simulink library "c166drivers"  (Simulink 6.0)
settings: Solver=ode45  SolverMode=SingleTasking  StartTime=0.0  StopTime=10.0  RelTol=1e-3
PreLoadFcn:
  | RTWConfigurationCB('preloadfcn', bdroot);
libraries: c166drivers x12, canblocks x8, exprofilelib x6, config_library x4, driver_interface_library x4, canblocks_extras x4, vector_candrivers x2, simulink x1
settings Model: Creator=The MathWorks Inc.  LastModifiedBy=batserve  ExtModeAutoUpdateStatusClock=off  ProdHWDeviceType=Specified
settings DataIOCC: SignalLoggingName=logsOut
settings OptimizationCC: BooleanDataType=off
settings DebuggingCC: CheckExecutionContextPreStartOutputMsg=on  CheckExecutionContextRuntimeOutputMsg=on  SolverPrmCheckMsg=none
settings HardwareCC: ProdHWDeviceType=Specified  TargetUnknown=on

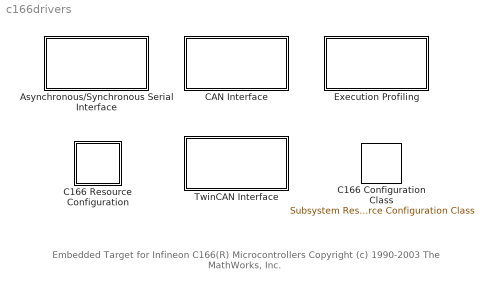
== system c166drivers ==
  note: Embedded Target for Infineon C166(R) Microcontrollers
      | Copyright (c) 1990-2003 The MathWorks, Inc.
  Asynchronous/Synchronous Serial Interface : Subsystem  PropExecContextAcrossSSBoundary=on
      mask Display: disp('Serial')
  C166 Configuration Class : config_library/Subsystem Resource Configuration Class  Tag=CONFIGURATION DATA CLASS  dClassName=c166Config.C166System  rClassName=c166Config.C166SystemResources
  C166 Resource Configuration : Subsystem  Tag=RTW CONFIGURATION BLOCK  AncestorBlock=|  PropExecContextAcrossSSBoundary=on  mask(Subsystem Resource Configuration){oldParentName=untitled2, oldBlockName=|, defaultConfigLibrary=}
      | config_library/Subsystem
      | Resource
      | Configuration
      mask oldBlockName=|
      | untitled2/C166
      | Resource
      | Configuration
      mask prompts: oldParentName "Old Parent Name"; oldBlockName "Old Block Name"; defaultConfigLibrary "Default Configuration Library"
      settings: CopyFcn=RTWConfigurationCB('copyfcn',gcb);  DeleteFcn=RTWConfigurationCB('deletefcn',gcb);  UndoDeleteFcn=RTWConfigurationCB('NameChangeFcn',gcb);  PreSaveFcn=RTWConfigurationCB('presavefcn',gcb);  NameChangeFcn=RTWConfigurationCB('NameChangeFcn',gcb);  OpenFcn=RTWConfigurationCB('openfcn',gcb);
      mask Display: image(imread('target_icon.jpg'))
  CAN Interface : Subsystem  PropExecContextAcrossSSBoundary=on
      mask Display: disp('CAN')
  Execution Profiling : Subsystem  PropExecContextAcrossSSBoundary=on
      mask Display: disp('Execution\nProfiling')
  TwinCAN Interface : Subsystem  PropExecContextAcrossSSBoundary=on
      mask Display: disp('TwinCAN')

== system c166drivers/Asynchronous/Synchronous Serial Interface ==
  ASC_Serial Configuration Class : config_library/Subsystem Resource Configuration Class  Tag=CONFIGURATION DATA CLASS  dClassName=c166Config.ASC_SERIAL  rClassName=""
  Serial Receive : S-Function  FunctionName=asc0_rx  Parameters=T,show_length,show_bytes_read, max_length  mask(C166 Serial Interface ASC0 Receive){show_length=on, show_bytes_read=on, max_length=1, T=1}
      mask prompts: show_length "Show input port for the requested number of bytes"; show_bytes_read "Show output port for the actual number of bytes read"; max_length "Maximum number of bytes:"; T "Sample time:"
      mask help: Receive bytes over the serial interface ASC0. Note that if the number of bytes available is smaller than the number of bytes requested then the actual number of bytes read is equal to the number of bytes available.
      mask init:
      | % Check for a C166 Resource Configuration block
      | target = RTWConfigurationCB('get_target', gcb);                            
      | target.checkName('C166');        
      | 
      | % Allocate the serial transmit interface
      | serial_interface = mask_resource_validator(gcb,@c166_serial_resource,'ASC0_RX');
      | if round(max_length)~=max_length | max_length<1
      | 	error('The maximum length of data parameter must be a positive integer')
      | end
      mask Help: helpview([docroot '/toolbox/c166/c166.map'], 'Serial_Receive');
      mask CallbackString:
      | s = get_param(gcb,'show_length');
      | if strcmp(s,'on')
      |    simUtil_maskParam('show',gcb,'max_length');
      | else
      |    simUtil_maskParam('hide',gcb,'max_length');
      | end
      | |||
      mask Display:
      | text(0.5, 0.5, 'ASC0\nReceive','horizontalAlignment','center')
      | port_label('output',1,'Data')
  Serial Transmit : S-Function  FunctionName=asc0_tx  Parameters=T,show_length,show_num_sent  mask(C166 Serial Interface ASC0 Transmit){show_length=on, show_num_sent=on, T=-1}
      mask prompts: show_length "Show input port for the number of bytes to transmit"; show_num_sent "Show output port for the actual number of bytes transmitted"; T "Sample time:"
      mask help: Transmit bytes over the serial interface ASC0. Note that if the number of available spaces in the buffer is smaller than the requested number of bytes to transmit then the actual number of bytes transmitted is equal to the number of spaces available.
      mask init:
      | % Check for a C166 Resource Configuration block
      | target = RTWConfigurationCB('get_target', gcb);                            
      | target.checkName('C166');        
      | 
      | % Allocate the serial transmit interface
      | serial_interface = mask_resource_validator(gcb,@c166_serial_resource,'ASC0_TX');
      mask Help: helpview([docroot '/toolbox/c166/c166.map'], 'Serial_Transmit');
      mask Display:
      | text(0.5, 0.5, 'ASC0\nTransmit','horizontalAlignment','center')
      | port_label('input',1,'Data')

== system c166drivers/C166 Resource Configuration ==
  config : S-Function  FunctionName=sfunRTWConfig

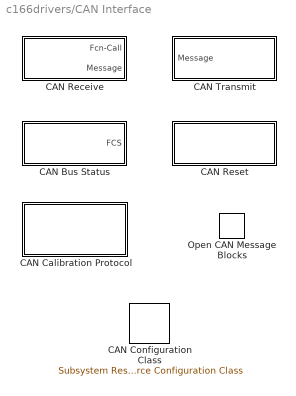
== system c166drivers/CAN Interface ==
  CAN Configuration Class : config_library/Subsystem Resource Configuration Class  Tag=CONFIGURATION DATA CLASS  dClassName=c166Config.CAN_C166  rClassName=c166Config.CAN_RESOURCES
  CAN Bus Status : Subsystem  PropExecContextAcrossSSBoundary=on  mask(C166 CAN Bus Status){module=A, status_type=Bus Off, t=1}
      mask prompts: status_type "Status type:"; t "Sample time:"
      mask help: Use this block to determine if the CAN controller is in either Bus Off state or Error Warning state.
      mask init:
      | dispstr = sprintf('CAN_%s\n%s Status', get_param(gcb,'module'),get_param(gcb,'status_type'));
      | 
      | % Check for a C166 Resource Configuration block
      | target = RTWConfigurationCB('get_target', gcb);                            
      | target.checkName('C166');        
      | 
      | if status_type == 1
      | 	status_str = 'Bus Off';
      | elseif status_type == 2
      | 	status_str = 'Error Warning';
      | end
      mask Help: helpview([docroot '/toolbox/c166/c166.map'], 'CAN_bus_status');
      mask StyleString: popup(A|B),popup(Bus Off|Error Warning),edit
      mask Display: disp(dispstr)
  CAN Calibration Protocol : Subsystem  TreatAsAtomicUnit=on  PropExecContextAcrossSSBoundary=on  mask(CAN Calibration Protocol (C166)){CCP_STATION_ID=hex2dec('1'), module=A, ccp_cro_id=hex2dec('6FA'), ccp_cro_message_type=Extended (29-bit identifier), ccp_return_id=hex2dec('6FB'), ccp_return_message_type=Extended (29-bit identifier), TOTAL_NUM_ODTS=8, cro_sample_time=0.01}
      mask prompts: CCP_STATION_ID "CCP station address (16-bit integer):"; module "CAN module:"; ccp_cro_id "CAN message identifier (CRO):"; ccp_cro_message_type "CAN message type (CRO):"; ccp_return_id "CAN message identifier (DTO/DAQ):"; ccp_return_message_type "CAN message type (DTO/DAQ):"; TOTAL_NUM_ODTS "Total Number of Object Descriptor Tables (ODTs):"; cro_sample_time "CRO sample time:"
      mask help:
      | Implements CAN Calibration Protocol (CCP v2.1) on the target processor.
      |
      | This block processes Command Receive Object (CRO) messages and outputs the resulting Data Transmission Object (DTO) and Data Acquisition (DAQ) messages.
      mask init:
      | % Propagate DTO message type to underlying blocks
      | set_param([gcb, '/DAQ Processing/Send DAQ Message/CAN Message Packing'], 'message_type', ccp_return_message_type);
      | set_param([gcb, '/DTO Processing/CCP (Termination)/CAN Transmit/DTO_Constructor'], 'message_type', ccp_return_message_type);
      | % Propagate CRO message type to underlying blocks
      | set_param([gcb, '/CAN Receive'], 'message_type', ccp_cro_message_type);
      | % Propagate CAN module to underlying blocks
      | set_param([gcb, '/DAQ Processing/Send DAQ Message/CAN Transmit'], 'module', module);
      | set_param([gcb, '/DTO Processing/CCP (Termination)/CAN Transmit/CAN Transmit'], 'module', module);
      | set_param([gcb, '/CAN Receive'], 'module', module);
      | 
      | % check for a Resource Config block, and make sure it is C166
      | target = RTWConfigurationCB('get_target', gcb);
      | target.checkName('C166');
      settings: CopyFcn=ccp_init_mask('copyfcn', gcb)
      mask Help: helpview([docroot '/toolbox/c166/c166.map'], 'target_CCP');
      mask StyleString: edit,popup(A|B),edit,popup(Standard (11-bit identifier)|Extended (29-bit identifier)),edit,popup(Standard (11-bit identifier)|Extended (29-bit identifier)),edit,edit
      mask Display: disp('CCP');
  CAN Receive : Subsystem  PropExecContextAcrossSSBoundary=on  mask(C166 CAN Receive){module=A, ids=hex2dec('0001'), buffer_select_mode=Automatic, bufferids=1, message_type=Standard (11-bit identifier), t=1}
      mask prompts: module "CAN module:"; ids "CAN message identifier:"; buffer_select_mode "Buffer selection:"; bufferids "Buffer number [1..15]:"; message_type "CAN message type:"; t "Sample time:"
      mask help: Receives CAN messages from the selected CAN module.
      mask init:
      | dispstr = sprintf('CAN_%s\nReceive',get_param(gcb,'module'));
      | 
      | % Check for a C166 Resource Configuration block
      | target = RTWConfigurationCB('get_target', gcb);                            
      | target.checkName('C166');        
      | 
      | if any(bufferids>15) | any(bufferids<1) | any( ~[bufferids==fix(bufferids)] )
      | 	error('Invalid CAN hardware buffer number specified. The buffer number number must be an integer in the range 1 to 15');
      | end
      | 
      | % Possibly auto-allocate the buffer
      | bufferids = mask_resource_validator(gcb,@c166_can_rx_validate, bufferids);
      | 
      | % check for valid CAN message identifier
      | can_msg_id_check(ids,message_type);
      | message_type=message_type-1;
      | 
      | % Check that module is enabled
      | c166_can_enabled_check(gcb,'CAN');
      mask Help: helpview([docroot '/toolbox/c166/c166.map'], 'CAN_RX');
      mask StyleString: popup(A|B),edit,popup(Automatic|Manual),edit,popup(Standard (11-bit identifier)|Extended (29-bit identifier)),edit
      mask CallbackString:
      | ||switch get_param(gcb,'buffer_select_mode');
      | 	case 'Automatic'
      | 		simUtil_maskParam('disable',gcb,'bufferids');
      | 	case 'Manual'
      |          simUtil_maskParam('enable',gcb,'bufferids');
      |  end
      |  |||
      mask Display:
      | disp(dispstr)
      | port_label('output',1,'f()');
      | port_label('output',2,'Msg');
  CAN Reset : Subsystem  PropExecContextAcrossSSBoundary=on  mask(C166 CAN Reset){module=A, t=-1}
      mask prompts: t "Sample time:"
      mask help: Place this block inside a triggered sub-system to reset the CAN module, for example, following entry to the Bus Off state.
      mask init:
      | dispstr = sprintf('CAN_%s\nReset', get_param(gcb,'module'));
      | 
      | % Check for a C166 Resource Configuration block
      | target = RTWConfigurationCB('get_target', gcb);                            
      | target.checkName('C166');
      mask Help: helpview([docroot '/toolbox/c166/c166.map'], 'CAN_reset');
      mask StyleString: popup(A|B),edit
      mask Display: disp(dispstr)
  CAN Transmit : Subsystem  PropExecContextAcrossSSBoundary=on  mask(C166 CAN Transmit){module=A, tx_mode=Queued transmission with shared buffer, fifo_queue_length=8, buffer_select_mode=Automatic, bufferids=1, t=-1, irq_level=0}
      mask prompts: tx_mode "Transmit mode:"; fifo_queue_length "Length (number of messages) of FIFO queue:"; buffer_select_mode "Buffer selection:"; bufferids "Buffer number [1..14]:"; t "Sample time:"; irq_level "Interrupt level (hidden)"
      mask help: Transmits a CAN message via the selected CAN module.
      mask init:
      | dispstr=sprintf('CAN_%s\nTransmit', get_param(gcb,'module'));
      | 
      | % Check for a C166 Resource Configuration block
      | target = RTWConfigurationCB('get_target', gcb);                            
      | target.checkName('C166');        
      | 
      | if bufferids==0 % special handling for un-initialized value
      | 	bufferids=1;
      | end
      | 
      | if any(bufferids>14) | any(bufferids<1) | any( ~[bufferids==fix(bufferids)] )
      | 	error('Invalid CAN hardware buffer number specified. The buffer number number must be an integer in the range 1 to 14 (it is not possible to use buffer 15 for transmit).');
      | end
      | 
      | 
      | % Check that module is enabled
      | c166_can_enabled_check(gcb,'CAN');
      | 
      | % Possibly auto-allocate the buffer
      | bufferids = mask_resource_validator(gcb,@c166_can_tx_validate,bufferids);
      | 
      | irq_level = 0;
      | 
      |   switch tx_mode
      |    case 1
      |     % no action
      |    case 2
      |     % no action
      |    case 3
      |     CAN = target.findConfigForClass('c166Config.CAN_C166');
      | 	if module == 1
      |         CAN.CAN_A.RequireIntDrivenFifoTx = 1;
      | 		irq_level = str2num(CAN.CAN_A.CAN_interrupt_level);
      | 	elseif module == 2
      |         CAN.CAN_B.RequireIntDrivenFifoTx = 1;
      | 		irq_level = str2num(CAN.CAN_B.CAN_Interrupt_Level);
      | 	end
      |    otherwise
      |     error('Invalid value for tx_mode')
      |   end
      mask Help: helpview([docroot '/toolbox/c166/c166.map'], 'CAN_TX');
      mask StyleString: popup(A|B),popup(Queued transmission with shared buffer|Direct transmission with dedicated buffer|FIFO queued transmission with dedicated buffer),edit,popup(Automatic|Manual),edit,edit,edit
      mask CallbackString:
      | |tempCanTxTxMode = get_param(gcb,'tx_mode');
      | switch tempCanTxTxMode
      | 	case {'Queued transmission with shared buffer'}
      | 		simUtil_maskParam('hide',gcb,'fifo_queue_length');
      | 		simUtil_maskParam('hide',gcb,'buffer_select_mode');
      | 		simUtil_maskParam('hide',gcb,'bufferids');
      | 	case {'Direct transmission with dedicated buffer'}
      | 		simUtil_maskParam('hide',gcb,'fifo_queue_length');
      | 		simUtil_maskParam('show',gcb,'buffer_select_mode');
      | 		simUtil_maskParam('show',gcb,'bufferids');
      |     case 'FIFO queued transmission with dedicated buffer'
      | 	    simUtil_maskParam('show',gcb,'fifo_queue_length');
      | 		simUtil_maskParam('show',gcb,'buffer_select_mode');
      | 		simUtil_maskParam('show',gcb,'bufferids');
      | 	otherwise
      | 		error(['Unrecognized value for tx_mode in ' gcb ]);
      | end
      | clear tempCanTxTxMode||switch get_param(gcb,'buffer_select_mode');
      | 	case 'Automatic'
      | 		simUtil_maskParam('disable',gcb,'bufferids');
      | 	case 'Manual'
      |          simUtil_maskParam('enable',gcb,'bufferids');
      |  end
      |  |
      |  ||
      mask Display:
      | disp(dispstr)
      | port_label('input',1,'Msg');
  Open CAN Message Blocks : vector_candrivers/Open CAN Message Blocks

== system c166drivers/Execution Profiling ==
  C166 Execution Profiling via ASC0 : Subsystem  TreatAsAtomicUnit=on  PropExecContextAcrossSSBoundary=on  mask(C166  Execution Profiling via Serial Port ASC0){t=1, execCopyFcn=on}
      mask prompts: t "Sample time:"; execCopyFcn "Execute CopyFcn"
      mask help:
      | Provides a serial interface to the execution profiling engine. On receipt of a start command to the serial port, logging of execution profile data begins. On completion of a logging run, the recorded data is automatically returned via serial.
      |
      | No other serial blocks may be used in the model if a C166 Execution Profiling via ASC0 block is present.
      |
      | See also the MATLAB command profile_c166.
      settings: CopyFcn=exprofile_copyfcn(gcb);
      mask Help: helpview([docroot '/toolbox/c166/c166.map'], 'Execution_Profiling_ASC0');
      mask Display: disp('Execution Profiling\nvia Serial')
  C166 Execution Profiling via CAN A : Subsystem  TreatAsAtomicUnit=on  PropExecContextAcrossSSBoundary=on  mask(C166 Execution Profiling via CAN Channel A){commandId=hex2dec('1FFFFF00'), dataId=hex2dec('1FFFFF01'), t=1, execCopyFcn=on}
      mask prompts: commandId "Start command CAN message identifier:"; dataId "Returned data CAN message identifier:"; t "Sample time:"; execCopyFcn "Execute CopyFcn"
      mask help:
      | Provides a CAN interface to the execution profiling engine. On receipt of a start command message, logging of execution profile data begins. On completion of a logging run, the recorded data is automatically returned via CAN.
      |
      | You must specify the message identifiers for the start command and the returned data. These identifiers must be compatible with the values used by the host-side part of the execution profiling utility. See also the MATLAB command profile_c166.
      settings: CopyFcn=exprofile_copyfcn(gcb);
      mask Help: helpview([docroot '/toolbox/c166/c166.map'], 'Execution_Profiling_Can_A');
      mask Display: disp('Execution Profiling\nvia CAN')
  C166 Execution Profiling via TwinCAN A : Subsystem  TreatAsAtomicUnit=on  PropExecContextAcrossSSBoundary=on  mask(C166 Execution Profiling via CAN Channel A){commandId=hex2dec('1FFFFF00'), dataId=hex2dec('1FFFFF01'), t=1, execCopyFcn=on}
      mask prompts: commandId "Start command CAN message identifier:"; dataId "Returned data CAN message identifier:"; t "Sample time:"; execCopyFcn "Execute CopyFcn"
      mask help:
      | Provides a CAN interface to the execution profiling engine. On receipt of a start command message, logging of execution profile data begins. On completion of a logging run, the recorded data is automatically returned via CAN.
      |
      | You must specify the message identifiers for the start command and the returned data. These identifiers must be compatible with the values used by the host-side part of the execution profiling utility. See also the MATLAB command profile_c166.
      settings: CopyFcn=exprofile_copyfcn(gcb);
      mask Help: helpview([docroot '/toolbox/c166/c166.map'], 'Execution_Profiling_Can_A');
      mask Display: disp('Execution Profiling\nvia CAN')

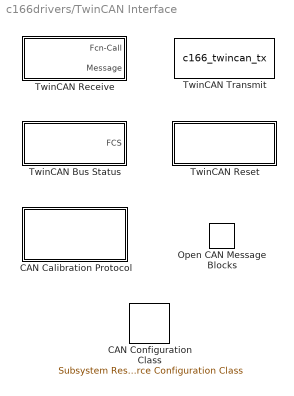
== system c166drivers/TwinCAN Interface ==
  CAN Configuration Class : config_library/Subsystem Resource Configuration Class  Tag=CONFIGURATION DATA CLASS  dClassName=c166Config.TwinCAN_C166  rClassName=c166Config.TwinCAN_RESOURCES
  CAN Calibration Protocol : Subsystem  TreatAsAtomicUnit=on  PropExecContextAcrossSSBoundary=on  mask(CAN Calibration Protocol (C166, TwinCAN)){CCP_STATION_ID=hex2dec('1'), module=A, ccp_cro_id=hex2dec('6FA'), ccp_cro_message_type=Extended (29-bit identifier), ccp_return_id=hex2dec('6FB'), ccp_return_message_type=Extended (29-bit identifier), TOTAL_NUM_ODTS=8, cro_sample_time=0.01}
      mask prompts: CCP_STATION_ID "CCP station address (16-bit integer):"; module "CAN module:"; ccp_cro_id "CAN message identifier (CRO):"; ccp_cro_message_type "CAN message type (CRO):"; ccp_return_id "CAN message identifier (DTO/DAQ):"; ccp_return_message_type "CAN message type (DTO/DAQ):"; TOTAL_NUM_ODTS "Total Number of Object Descriptor Tables (ODTs):"; cro_sample_time "CRO sample time:"
      mask help:
      | Implements CAN Calibration Protocol (CCP v2.1) on the target processor with TwinCAN module.
      |
      | This block processes Command Receive Object (CRO) messages and outputs the resulting Data Transmission Object (DTO) and Data Acquisition (DAQ) messages.
      mask init: same as c166drivers/CAN Interface/CAN Calibration Protocol
      settings: CopyFcn=ccp_init_mask('copyfcn', gcb)
      mask Help: helpview([docroot '/toolbox/c166/c166.map'], 'TWINCAN_target_CCP');
      mask StyleString: edit,popup(A|B),edit,popup(Standard (11-bit identifier)|Extended (29-bit identifier)),edit,popup(Standard (11-bit identifier)|Extended (29-bit identifier)),edit,edit
      mask Display: disp('CCP\n(TwinCAN)');
  Open CAN Message Blocks : vector_candrivers/Open CAN Message Blocks
  TwinCAN Bus Status : Subsystem  PropExecContextAcrossSSBoundary=on  mask(C166 TwinCAN Bus Status){module=A, status_type=Bus Off, t=1}
      mask prompts: module "TwinCAN node:"; status_type "Status type:"; t "Sample time:"
      mask help: Use this block to determine if the CAN controller is in either Bus Off state or Error Warning state.
      mask init:
      | dispstr = sprintf('TwinCAN_%s\n%s Status', get_param(gcb,'module'),get_param(gcb,'status_type'));
      | 
      | % Check for a C166 Resource Configuration block
      | target = RTWConfigurationCB('get_target', gcb);                            
      | target.checkName('C166');        
      | 
      | if status_type == 1
      | 	status_str = 'Bus Off';
      | elseif status_type == 2
      | 	status_str = 'Error Warning';
      | end
      mask Help: helpview([docroot '/toolbox/c166/c166.map'], 'TWINCAN_bus_status');
      mask StyleString: popup(A|B),popup(Bus Off|Error Warning),edit
      mask Display: disp(dispstr)
  TwinCAN Receive : Subsystem  PropExecContextAcrossSSBoundary=on  mask(C166 TwinCAN Receive){module=A, ids=hex2dec('0001'), message_type=Standard (11-bit identifier), bufferids=0, t=1}
      mask prompts: module "TwinCAN node:"; ids "CAN message identifier:"; message_type "CAN message type:"; bufferids "Buffers (hidden)"; t "Sample time:"
      mask help: Receives CAN messages from the selected TwinCAN module.
      mask init:
      | dispstr = sprintf('TwinCAN_%s\nReceive',get_param(gcb,'module'));
      | 
      | % Check for a C166 Resource Configuration block
      | target = RTWConfigurationCB('get_target', gcb);                            
      | target.checkName('C166');        
      | 
      | % Auto-allocate the buffer
      | bufferids = mask_resource_validator(gcb,@c166_twincan_rx_validate, bufferids);
      | 
      | % Check for valid CAN message identifier
      | can_msg_id_check(ids,message_type);
      | message_type=message_type-1;
      | 
      | % Check that module is enabled
      | c166_can_enabled_check(gcb,'TwinCAN');
      mask Help: helpview([docroot '/toolbox/c166/c166.map'], 'TWINCAN_RX');
      mask StyleString: popup(A|B),edit,popup(Standard (11-bit identifier)|Extended (29-bit identifier)),edit,edit
      mask Display:
      | disp(dispstr)
      | port_label('output',1,'f()');
      | port_label('output',2,'Msg');
  TwinCAN Reset : Subsystem  PropExecContextAcrossSSBoundary=on  mask(C166 TwinCAN Reset){t=-1}
      mask prompts: t "Sample time:"
      mask help: Place this block inside a triggered sub-system to reset the TwinCAN module, for example, following entry of one of the nodes into Bus Off state.
      mask init:
      | dispstr = sprintf('TwinCAN\nReset');
      | 
      | % Check for a C166 Resource Configuration block
      | target = RTWConfigurationCB('get_target', gcb);                            
      | target.checkName('C166');
      mask Help: helpview([docroot '/toolbox/c166/c166.map'], 'TWINCAN_reset');
      mask Display: disp(dispstr)
  TwinCAN Transmit : S-Function  FunctionName=c166_twincan_tx  Parameters=module, tx_mode, fifo_queue_length, uint32(bufferids), irq_level, t  mask(C166 TwinCAN Transmit){module=A, tx_mode=Direct transmission with dedicated buffer, fifo_queue_length=8, buffer_select_mode=Automatic, bufferids=0, t=-1, irq_level=0}
      mask prompts: module "TwinCAN Node:"; tx_mode "Transmit mode:"; fifo_queue_length "Length (number of messages) of FIFO queue:"; buffer_select_mode "Buffer selection:"; bufferids "Buffer number [0..31]:"; t "Sample time:"; irq_level "Interrupt Level (hidden):"
      mask help: Transmits a CAN message via the selected TwinCAN module.
      mask init:
      | dispstr=sprintf('TwinCAN_%s\nTransmit', get_param(gcb,'module'));
      | 
      | % Check for a C166 Resource Configuration block
      | target = RTWConfigurationCB('get_target', gcb);                            
      | target.checkName('C166');        
      | 
      | if any(bufferids>31) | any(bufferids<0) | any( ~[bufferids==fix(bufferids)] )
      | 	error('Invalid CAN hardware buffer number specified. The buffer number number must be an integer in the range 0 to 31');
      | end
      | 
      | % Check that module is enabled
      | c166_can_enabled_check(gcb,'TwinCAN');
      | 
      | % Auto-allocate the buffer
      | bufferids = mask_resource_validator(gcb,@c166_twincan_tx_validate,bufferids);
      | 
      | irq_level = 0;
      | 
      | % Register any requirement to use interrupt driven FIFO transmit
      |   switch tx_mode
      |    case 1
      |     % no action
      |    case 2
      |     twinCAN = target.findConfigForClass('c166Config.TwinCAN_C166');
      | 	if module == 1
      |         twinCAN.CAN_A.RequireIntDrivenFifoTx = 1;
      | 		irq_level = str2num(twinCAN.CAN_A.CAN_Interrupt_Level);
      | 	elseif module == 2
      |         twinCAN.CAN_B.RequireIntDrivenFifoTx = 1;
      | 		irq_level = str2num(twinCAN.CAN_B.CAN_Interrupt_Level);
      | 	end
      |    otherwise
      |     error('Invalid value for tx_mode')
      |   end
      mask Help: helpview([docroot '/toolbox/c166/c166.map'], 'TWINCAN_TX');
      mask StyleString: popup(A|B),popup(Direct transmission with dedicated buffer|FIFO queued transmission with dedicated buffer),edit,popup(Automatic|Manual),edit,edit,edit
      mask CallbackString:
      | |tempCanTxTxMode = get_param(gcb,'tx_mode');
      | switch tempCanTxTxMode
      | 	case {'Direct transmission with dedicated buffer'}
      | 		simUtil_maskParam('hide',gcb,'fifo_queue_length');
      |     case 'FIFO queued transmission with dedicated buffer'
      | 	    simUtil_maskParam('show',gcb,'fifo_queue_length');
      | 	otherwise
      | 		error(['Unrecognized value for tx_mode in ' gcb ]);
      | end
      | clear tempCanTxTxMode||switch get_param(gcb,'buffer_select_mode');
      | 	case 'Automatic'
      | 		simUtil_maskParam('disable',gcb,'bufferids');
      | 	case 'Manual'
      |          simUtil_maskParam('enable',gcb,'bufferids');
      |  end
      |  |||
      mask Display:
      | disp(dispstr)
      | port_label('input',1,'Msg');

== system c166drivers/CAN Interface/CAN Bus Status ==
  can_status : S-Function  FunctionName=c166_can_status  Parameters=module, status_str, t
  FCS : Outport
  wires:
  can_status/1 -> FCS/1

== system c166drivers/CAN Interface/CAN Calibration Protocol ==
  CAN Receive : c166drivers/CAN Interface/CAN Receive  module=A  ids=ccp_cro_id  buffer_select_mode=Automatic  bufferids=1  message_type=Extended (29-bit identifier)  t=cro_sample_time
  DAQ Processing : Subsystem  PropExecContextAcrossSSBoundary=on
      mask Display: disp('DAQ');
  DTO Processing : Subsystem  TreatAsAtomicUnit=on  PropExecContextAcrossSSBoundary=on
      mask Display: disp('DTO');
  wires:
  CAN Receive/1 -> DTO Processing/Trigger
  CAN Receive/2 -> DTO Processing/1(CRO)

== system c166drivers/CAN Interface/CAN Receive ==
  CAN Receive (S-Function) : S-Function  FunctionName=c166_can_rx  Parameters=module uint32(ids) t message_type uint32(bufferids)
  Fcn-Call : Outport
  Message : Outport  Port=2
  wires:
  CAN Receive (S-Function)/1 -> Fcn-Call/1  "Fcn-Call (real-time)"
  CAN Receive (S-Function)/2 -> Message/1  "Data (real-time)"

== system c166drivers/CAN Interface/CAN Reset ==
  can_reset : S-Function  FunctionName=c166_can_reset  Parameters=module, t

== system c166drivers/CAN Interface/CAN Transmit ==
  Message : Inport  Port=1  LatchInput=off
  CAN Transmit : S-Function  FunctionName=c166_can_tx  Parameters=module, tx_mode, uint32(bufferids), fifo_queue_length, irq_level, t
  wires:
  Message/1 -> CAN Transmit/1

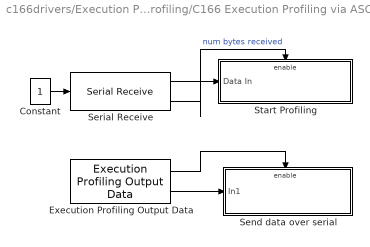
== system c166drivers/Execution Profiling/C166 Execution Profiling via ASC0 ==
  Constant : Constant  OutDataTypeMode=uint8
  Execution Profiling Output Data : exprofilelib/Execution Profiling Output Data  t=t
  Send data over serial : Subsystem  TreatAsAtomicUnit=on  PropExecContextAcrossSSBoundary=on
  Serial Receive : c166drivers/Asynchronous//Synchronous Serial Interface/Serial Receive  show_length=on  show_bytes_read=on  max_length=1  T=t
  Start Profiling : Subsystem  PropExecContextAcrossSSBoundary=on
  wires:
  Serial Receive/2 -> Start Profiling/Enable  "num bytes received"
  Serial Receive/1 -> Start Profiling/1(Data In)
  Constant/1 -> Serial Receive/1
  Execution Profiling Output Data/1 -> Send data over serial/Enable
  Execution Profiling Output Data/2 -> Send data over serial/1(In1)

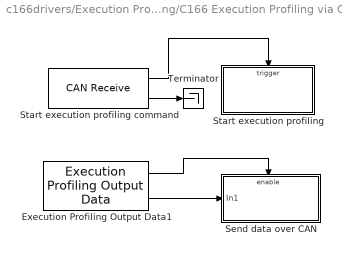
== system c166drivers/Execution Profiling/C166 Execution Profiling via CAN A ==
  Execution Profiling Output Data1 : exprofilelib/Execution Profiling Output Data  t=t
  Send data over CAN : Subsystem  TreatAsAtomicUnit=on  PropExecContextAcrossSSBoundary=on
  Start execution profiling : Subsystem  PropExecContextAcrossSSBoundary=on
  Start execution profiling command : c166drivers/CAN Interface/CAN Receive  module=A  ids=commandId  buffer_select_mode=Automatic  bufferids=2  message_type=Extended (29-bit identifier)  t=t
  Terminator : Terminator
  wires:
  Start execution profiling command/2 -> Terminator/1
  Start execution profiling command/1 -> Start execution profiling/Trigger
  Execution Profiling Output Data1/1 -> Send data over CAN/Enable
  Execution Profiling Output Data1/2 -> Send data over CAN/1(In1)

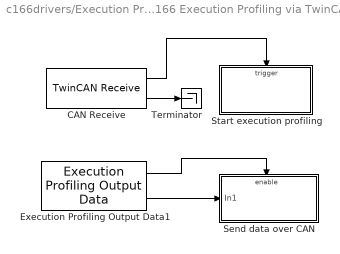
== system c166drivers/Execution Profiling/C166 Execution Profiling via TwinCAN A ==
  CAN Receive : c166drivers/TwinCAN Interface/TwinCAN Receive  module=A  ids=commandId  message_type=Extended (29-bit identifier)  bufferids=0  t=t
  Execution Profiling Output Data1 : exprofilelib/Execution Profiling Output Data  t=t
  Send data over CAN : Subsystem  TreatAsAtomicUnit=on  PropExecContextAcrossSSBoundary=on
  Start execution profiling : Subsystem  PropExecContextAcrossSSBoundary=on
  Terminator : Terminator
  wires:
  Execution Profiling Output Data1/2 -> Send data over CAN/1(In1)
  Execution Profiling Output Data1/1 -> Send data over CAN/Enable
  CAN Receive/1 -> Start execution profiling/Trigger
  CAN Receive/2 -> Terminator/1

== system c166drivers/TwinCAN Interface/CAN Calibration Protocol ==
  CAN Receive : c166drivers/TwinCAN Interface/TwinCAN Receive  module=A  ids=ccp_cro_id  message_type=Extended (29-bit identifier)  bufferids=0  t=cro_sample_time
  DAQ Processing : Subsystem  PropExecContextAcrossSSBoundary=on
      mask Display: disp('DAQ');
  DTO Processing : Subsystem  TreatAsAtomicUnit=on  PropExecContextAcrossSSBoundary=on
      mask Display: disp('DTO');
  wires:
  CAN Receive/1 -> DTO Processing/Trigger
  CAN Receive/2 -> DTO Processing/1(CRO)

== system c166drivers/TwinCAN Interface/TwinCAN Bus Status ==
  can_status : S-Function  FunctionName=c166_twincan_status  Parameters=module, status_str, t
  FCS : Outport
  wires:
  can_status/1 -> FCS/1

== system c166drivers/TwinCAN Interface/TwinCAN Receive ==
  TwinCAN Receive (S-Function) : S-Function  FunctionName=c166_twincan_rx  Parameters=module uint32(ids) t message_type uint32(bufferids)
  Fcn-Call : Outport
  Message : Outport  Port=2
  wires:
  TwinCAN Receive (S-Function)/2 -> Message/1  "Data (real-time)"
  TwinCAN Receive (S-Function)/1 -> Fcn-Call/1  "Fcn-Call (real-time)"

== system c166drivers/TwinCAN Interface/TwinCAN Reset ==
  can_reset : S-Function  FunctionName=c166_twincan_reset  Parameters=t

== system c166drivers/CAN Interface/CAN Calibration Protocol/DAQ Processing ==
  note: Must use "RTW memory get" block to access the msg_pointer
  Function Definition : driver_interface_library/Function Definition  function_name='void exported_ccp_daq_trigger(uint8_T * msg_pointer)'
  Send DAQ Message : Subsystem  TreatAsAtomicUnit=on  PropExecContextAcrossSSBoundary=on
      mask Type: Send DAQ Message
  wires:
  Function Definition/1 -> Send DAQ Message/Trigger

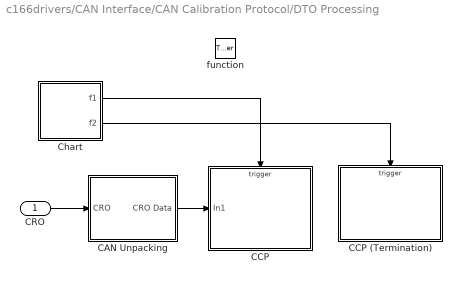
== system c166drivers/CAN Interface/CAN Calibration Protocol/DTO Processing ==
  CRO : Inport  Port=1  LatchInput=off
  function : TriggerPort  TriggerType=function-call
  CAN Unpacking : Subsystem  PropExecContextAcrossSSBoundary=on
  CCP : Subsystem  TreatAsAtomicUnit=on  PropExecContextAcrossSSBoundary=on
      mask Type: CCP
  CCP (Termination) : Subsystem  TreatAsAtomicUnit=on  PropExecContextAcrossSSBoundary=on
      mask Type: CCP (Termination)
  Chart : Stateflow chart  PropExecContextAcrossSSBoundary=on
  wires:
  CRO/1 -> CAN Unpacking/1(CRO)
  Chart/2(f2) -> CCP (Termination)/Trigger
  CAN Unpacking/1(CRO Data) -> CCP/1(In1)
  Chart/1(f1) -> CCP/Trigger

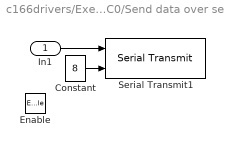
== system c166drivers/Execution Profiling/C166 Execution Profiling via ASC0/Send data over serial ==
  In1 : Inport  Port=1  LatchInput=off
  Enable : EnablePort
  Constant : Constant  Value=8  OutDataTypeMode=uint8
  Serial Transmit1 : c166drivers/Asynchronous//Synchronous Serial Interface/Serial Transmit  show_length=on  show_num_sent=off  T=-1
  wires:
  In1/1 -> Serial Transmit1/1
  Constant/1 -> Serial Transmit1/2

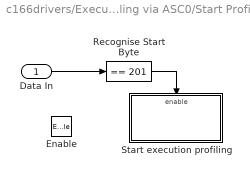
== system c166drivers/Execution Profiling/C166 Execution Profiling via ASC0/Start Profiling ==
  Data In : Inport  Port=1  LatchInput=off
  Enable : EnablePort
  Recognise Start Byte : simulink/Logic and Bit Operations/Compare To Constant  relop===  const=201  LogicOutDataTypeMode=uint8
  Start execution profiling : Subsystem  PropExecContextAcrossSSBoundary=on
  wires:
  Data In/1 -> Recognise Start Byte/1
  Recognise Start Byte/1 -> Start execution profiling/Enable

== system c166drivers/Execution Profiling/C166 Execution Profiling via CAN A/Send data over CAN ==
  In1 : Inport  Port=1  LatchInput=off
  Enable : EnablePort
  CAN Message Packing : canblocks/CAN Message Packing  id=dataId  message_type=Extended (29-bit identifier)  endian=Little Endian (Intel)
  CAN Transmit : c166drivers/CAN Interface/CAN Transmit  module=A  tx_mode=FIFO queued transmission with dedicated buffer  fifo_queue_length=8  buffer_select_mode=Automatic  bufferids=0  t=-1  irq_level=0
  wires:
  CAN Message Packing/1 -> CAN Transmit/1
  In1/1 -> CAN Message Packing/1

== system c166drivers/Execution Profiling/C166 Execution Profiling via CAN A/Start execution profiling ==
  function : TriggerPort  TriggerType=function-call  ZeroCross=off
  Execution Profiling Start : exprofilelib/Execution Profiling Start

== system c166drivers/Execution Profiling/C166 Execution Profiling via TwinCAN A/Send data over CAN ==
  In1 : Inport  Port=1  LatchInput=off
  Enable : EnablePort
  CAN Message Packing : canblocks/CAN Message Packing  id=dataId  message_type=Extended (29-bit identifier)  endian=Little Endian (Intel)
  CAN Transmit : c166drivers/TwinCAN Interface/TwinCAN Transmit  module=A  tx_mode=FIFO queued transmission with dedicated buffer  fifo_queue_length=8  buffer_select_mode=Manual  bufferids=28  t=-1  irq_level=0
  wires:
  In1/1 -> CAN Message Packing/1
  CAN Message Packing/1 -> CAN Transmit/1

== system c166drivers/Execution Profiling/C166 Execution Profiling via TwinCAN A/Start execution profiling ==
  function : TriggerPort  TriggerType=function-call  ZeroCross=off
  Execution Profiling Start : exprofilelib/Execution Profiling Start

== system c166drivers/TwinCAN Interface/CAN Calibration Protocol/DAQ Processing ==
  note: Must use "RTW memory get" block to access the msg_pointer
  Function Definition : driver_interface_library/Function Definition  function_name='void exported_ccp_daq_trigger(uint8_T * msg_pointer)'
  Send DAQ Message : Subsystem  TreatAsAtomicUnit=on  PropExecContextAcrossSSBoundary=on
      mask Type: Send DAQ Message
  wires:
  Function Definition/1 -> Send DAQ Message/Trigger

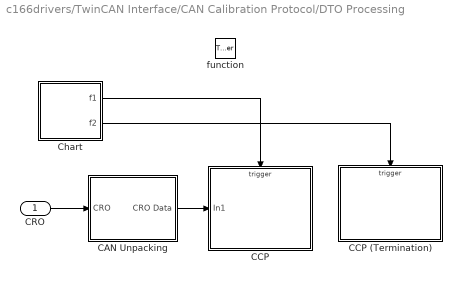
== system c166drivers/TwinCAN Interface/CAN Calibration Protocol/DTO Processing ==
  CRO : Inport  Port=1  LatchInput=off
  function : TriggerPort  TriggerType=function-call
  CAN Unpacking : Subsystem  PropExecContextAcrossSSBoundary=on
  CCP : Subsystem  TreatAsAtomicUnit=on  PropExecContextAcrossSSBoundary=on
      mask Type: CCP
  CCP (Termination) : Subsystem  TreatAsAtomicUnit=on  PropExecContextAcrossSSBoundary=on
      mask Type: CCP (Termination)
  Chart : Stateflow chart  PropExecContextAcrossSSBoundary=on
  wires:
  CRO/1 -> CAN Unpacking/1(CRO)
  Chart/2(f2) -> CCP (Termination)/Trigger
  CAN Unpacking/1(CRO Data) -> CCP/1(In1)
  Chart/1(f1) -> CCP/Trigger

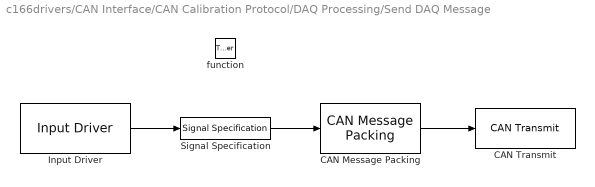
== system c166drivers/CAN Interface/CAN Calibration Protocol/DAQ Processing/Send DAQ Message ==
  function : TriggerPort  TriggerType=function-call
  CAN Message Packing : canblocks/CAN Message Packing  id=ccp_return_id  message_type=Extended (29-bit identifier)  endian=Little Endian (Intel)
  CAN Transmit : c166drivers/CAN Interface/CAN Transmit  module=A  tx_mode=FIFO queued transmission with dedicated buffer  fifo_queue_length=8  buffer_select_mode=Automatic  bufferids=0  t=-1  irq_level=0
  Input Driver : driver_interface_library/Input Driver  t=-1  expr='msg_pointer[%<i>]'  portWidth=8  pOpt=[]  expression_type=Not expression
  Signal Specification : SignalSpecification  DataType=uint8
  wires:
  Signal Specification/1 -> CAN Message Packing/1
  Input Driver/1 -> Signal Specification/1
  CAN Message Packing/1 -> CAN Transmit/1

== system c166drivers/CAN Interface/CAN Calibration Protocol/DTO Processing/CAN Unpacking ==
  CRO : Inport  Port=1  LatchInput=off
  CAN Message Unpacking : canblocks/CAN Message Unpacking/CAN Message Unpacking  showData=on  showID=off  showLength=off  endian=Little Endian (Intel)
  Signal Specification : SignalSpecification  Dimensions=8  DataType=uint8
  CRO Data : Outport
  wires:
  Signal Specification/1 -> CRO Data/1
  CRO/1 -> CAN Message Unpacking/1
  CAN Message Unpacking/1 -> Signal Specification/1

== system c166drivers/CAN Interface/CAN Calibration Protocol/DTO Processing/CCP ==
  In1 : Inport  Port=1  LatchInput=off
  function : TriggerPort  TriggerType=function-call
  CAN Calibration Protocol : canblocks_extras/CAN Calibration Protocol  CCP_STATION_ID=CCP_STATION_ID  TOTAL_NUM_ODTS=TOTAL_NUM_ODTS  show_commands=off  GET_CCP_VERSIONenabled=on  EXCHANGE_IDenabled=on  SET_MTAenabled=on  DNLOADenabled=on  DNLOAD_6enabled=on  UPLOADenabled=on  SHORT_UPenabled=on  GET_DAQ_SIZEenabled=on  SET_DAQ_PTRenabled=on  WRITE_DAQenabled=on  START_STOPenabled=on  SET_S_STATUSenabled=on  GET_S_STATUSenabled=on  START_STOP_ALLenabled=on
      settings: AttributesFormatString=\n\n
  wires:
  In1/1 -> CAN Calibration Protocol/1

== system c166drivers/CAN Interface/CAN Calibration Protocol/DTO Processing/CCP (Termination) ==
  function : TriggerPort  TriggerType=function-call
  CAN Calibration Protocol (Termination) : canblocks_extras/CAN Calibration Protocol (Termination)
      settings: AttributesFormatString=\n\n
  CAN Transmit : Subsystem  TreatAsAtomicUnit=on  PropExecContextAcrossSSBoundary=on
      mask Type: CAN Transmit
  wires:
  CAN Calibration Protocol (Termination)/1 -> CAN Transmit/Trigger
  CAN Calibration Protocol (Termination)/2 -> CAN Transmit/1(DTO Data)

== system c166drivers/Execution Profiling/C166 Execution Profiling via ASC0/Start Profiling/Start execution profiling ==
  Enable : EnablePort
  Execution Profiling Start : exprofilelib/Execution Profiling Start

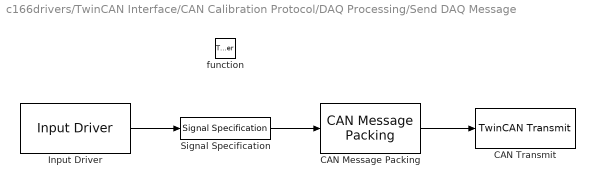
== system c166drivers/TwinCAN Interface/CAN Calibration Protocol/DAQ Processing/Send DAQ Message ==
  function : TriggerPort  TriggerType=function-call
  CAN Message Packing : canblocks/CAN Message Packing  id=ccp_return_id  message_type=Extended (29-bit identifier)  endian=Little Endian (Intel)
  CAN Transmit : c166drivers/TwinCAN Interface/TwinCAN Transmit  module=A  tx_mode=FIFO queued transmission with dedicated buffer  fifo_queue_length=8  buffer_select_mode=Automatic  bufferids=0  t=-1  irq_level=0
  Input Driver : driver_interface_library/Input Driver  t=-1  expr='msg_pointer[%<i>]'  portWidth=8  pOpt=[]  expression_type=Not expression
  Signal Specification : SignalSpecification  DataType=uint8
  wires:
  Signal Specification/1 -> CAN Message Packing/1
  Input Driver/1 -> Signal Specification/1
  CAN Message Packing/1 -> CAN Transmit/1

== system c166drivers/TwinCAN Interface/CAN Calibration Protocol/DTO Processing/CAN Unpacking ==
  CRO : Inport  Port=1  LatchInput=off
  CAN Message Unpacking : canblocks/CAN Message Unpacking/CAN Message Unpacking  showData=on  showID=off  showLength=off  endian=Little Endian (Intel)
  Signal Specification : SignalSpecification  Dimensions=8  DataType=uint8
  CRO Data : Outport
  wires:
  Signal Specification/1 -> CRO Data/1
  CRO/1 -> CAN Message Unpacking/1
  CAN Message Unpacking/1 -> Signal Specification/1

== system c166drivers/TwinCAN Interface/CAN Calibration Protocol/DTO Processing/CCP ==
  In1 : Inport  Port=1  LatchInput=off
  function : TriggerPort  TriggerType=function-call
  CAN Calibration Protocol : canblocks_extras/CAN Calibration Protocol  CCP_STATION_ID=CCP_STATION_ID  TOTAL_NUM_ODTS=TOTAL_NUM_ODTS  show_commands=off  GET_CCP_VERSIONenabled=on  EXCHANGE_IDenabled=on  SET_MTAenabled=on  DNLOADenabled=on  DNLOAD_6enabled=on  UPLOADenabled=on  SHORT_UPenabled=on  GET_DAQ_SIZEenabled=on  SET_DAQ_PTRenabled=on  WRITE_DAQenabled=on  START_STOPenabled=on  SET_S_STATUSenabled=on  GET_S_STATUSenabled=on  START_STOP_ALLenabled=on
      settings: AttributesFormatString=\n\n
  wires:
  In1/1 -> CAN Calibration Protocol/1

== system c166drivers/TwinCAN Interface/CAN Calibration Protocol/DTO Processing/CCP (Termination) ==
  function : TriggerPort  TriggerType=function-call
  CAN Calibration Protocol (Termination) : canblocks_extras/CAN Calibration Protocol (Termination)
      settings: AttributesFormatString=\n\n
  CAN Transmit : Subsystem  TreatAsAtomicUnit=on  PropExecContextAcrossSSBoundary=on
      mask Type: CAN Transmit
  wires:
  CAN Calibration Protocol (Termination)/1 -> CAN Transmit/Trigger
  CAN Calibration Protocol (Termination)/2 -> CAN Transmit/1(DTO Data)

== system c166drivers/CAN Interface/CAN Calibration Protocol/DTO Processing/CCP (Termination)/CAN Transmit ==
  DTO Data : Inport  Port=1  LatchInput=off
  function : TriggerPort  TriggerType=function-call
  CAN Transmit : c166drivers/CAN Interface/CAN Transmit  module=A  tx_mode=Queued transmission with shared buffer  fifo_queue_length=8  buffer_select_mode=Automatic  bufferids=0  t=-1  irq_level=0
  DTO_Constructor : canblocks/CAN Message Packing  id=ccp_return_id  message_type=Extended (29-bit identifier)  endian=Little Endian (Intel)
  wires:
  DTO Data/1 -> DTO_Constructor/1
  DTO_Constructor/1 -> CAN Transmit/1

== system c166drivers/TwinCAN Interface/CAN Calibration Protocol/DTO Processing/CCP (Termination)/CAN Transmit ==
  DTO Data : Inport  Port=1  LatchInput=off
  function : TriggerPort  TriggerType=function-call
  CAN Transmit : c166drivers/TwinCAN Interface/TwinCAN Transmit  module=A  tx_mode=Direct transmission with dedicated buffer  fifo_queue_length=8  buffer_select_mode=Automatic  bufferids=0  t=-1  irq_level=0
  DTO_Constructor : canblocks/CAN Message Packing  id=ccp_return_id  message_type=Extended (29-bit identifier)  endian=Little Endian (Intel)
  wires:
  DTO Data/1 -> DTO_Constructor/1
  DTO_Constructor/1 -> CAN Transmit/1

== stateflow chart TwinCAN Interface/CAN Calibration Protocol/DTO Processing/Chart ==
  (default) -> (junction 3) : {f1;f2;}
  events: f1 output FUNCTION_CALL_EVENT; f2 output FUNCTION_CALL_EVENT

== stateflow chart CAN Interface/CAN Calibration Protocol/DTO Processing/Chart ==
  (default) -> (junction 9) : {f1;f2;}
  events: f1 output FUNCTION_CALL_EVENT; f2 output FUNCTION_CALL_EVENT
